simulink model "ABAG"  (R2015a)
settings: Solver=ode3  StartTime=0.0  StopTime=10.0  FixedStep=0.1  RelTol=1e-3
libraries: simulink x1
settings Model: Creator=s141010  LastModifiedBy=s141010

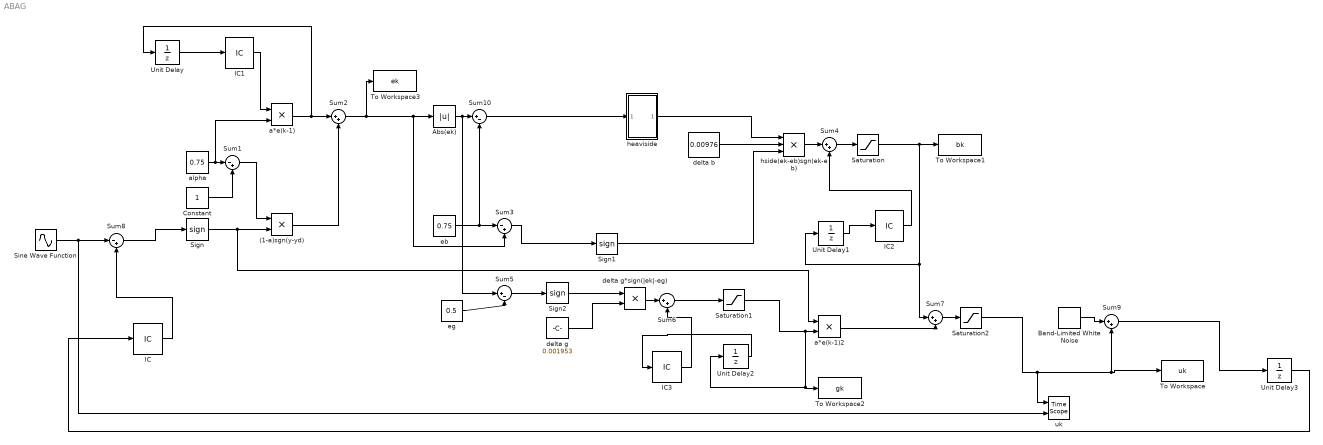
== system ABAG ==
  (1-a)sgn(y-yd) : Product
  Abs(ek) : Abs
  Band-Limited White Noise : simulink/Sources/Band-Limited White Noise  Cov=[0.1]  Ts=0.1  seed=[23341]
  Constant : Constant
  IC{,1..3} (4 alike) : InitialCondition
  Saturation : Saturate  UpperLimit=1  LowerLimit=0
  Saturation1 : Saturate  UpperLimit=1  LowerLimit=0
  Saturation2 : Saturate  UpperLimit=1  LowerLimit=0
  Sign : Signum
  Sign1 : Signum
  Sign2 : Signum
  Sine Wave Function : Sin  SampleTime=0.1
  Sum1 : Sum  Inputs=|-+
  Sum10 : Sum  Inputs=|+-
  Sum{2,4,6..7,9} (5 alike) : Sum  Inputs=|++
  Sum3 : Sum  Inputs=|-+
  Sum5 : Sum  Inputs=|+-
  Sum8 : Sum  Inputs=|-+
  To Workspace : ToWorkspace  VariableName=uk  SampleTime=-1
  To Workspace1 : ToWorkspace  VariableName=bk  SampleTime=-1
  To Workspace2 : ToWorkspace  VariableName=gk  SampleTime=-1
  To Workspace3 : ToWorkspace  VariableName=ek  SampleTime=-1
  Unit Delay : UnitDelay  InputProcessing=Columns as channels (frame based)  SampleTime=-1
  Unit Delay1 : UnitDelay  SampleTime=-1
  Unit Delay2 : UnitDelay  InputProcessing=Columns as channels (frame based)  SampleTime=-1
  Unit Delay3 : UnitDelay  SampleTime=-1
  a*e(k-1) : Product
  a*e(k-1)2 : Product
  alpha : Constant  Value=0.75
  delta b : Constant  Value=0.00976
  delta g : Constant  Value=0.001953
  delta g*sign(|ek|-eg) : Product
  eb : Constant  Value=0.75
  eg : Constant  Value=0.5
  heaviside : Subsystem
  hside(ek-eb)sgn(ek-eb) : Product  Inputs=3
  uk : TimeScope  NumInputPorts=2
  wires:
  Sign/1 -> a*e(k-1)2/1, (1-a)sgn(y-yd)/2
  Sum1/1 -> (1-a)sgn(y-yd)/1
  Constant/1 -> Sum1/2
  alpha/1 -> a*e(k-1)/2, Sum1/1
  (1-a)sgn(y-yd)/1 -> Sum2/2
  Sum2/1 -> To Workspace3/1, Abs(ek)/1, Sum3/2
  eb/1 -> Sum3/1, Sum10/2
  hside(ek-eb)sgn(ek-eb)/1 -> Sum4/1
  Saturation/1 -> To Workspace1/1, Sum7/1, Unit Delay1/1
  Sum3/1 -> Sign1/1
  eg/1 -> Sum5/2
  Sum5/1 -> Sign2/1
  Sign2/1 -> delta g*sign(|ek|-eg)/1
  delta g/1 -> delta g*sign(|ek|-eg)/2
  Unit Delay2/1 -> IC3/1
  delta g*sign(|ek|-eg)/1 -> Sum6/1
  Sine Wave Function/1 -> uk/2, Sum8/1
  Unit Delay3/1 -> IC/1
  Sum8/1 -> Sign/1
  Band-Limited White Noise/1 -> Sum9/1
  Sum9/1 -> Unit Delay3/1
  Sum4/1 -> Saturation/1
  Saturation1/1 -> Unit Delay2/1, To Workspace2/1, a*e(k-1)2/2
  Sum6/1 -> Saturation1/1
  Sum7/1 -> Saturation2/1
  Saturation2/1 -> To Workspace/1, Sum9/2, uk/1
  a*e(k-1)2/1 -> Sum7/2
  Sign1/1 -> hside(ek-eb)sgn(ek-eb)/3
  Abs(ek)/1 -> Sum5/1, Sum10/1
  a*e(k-1)/1 -> Unit Delay/1, Sum2/1
  Unit Delay1/1 -> IC2/1
  Sum10/1 -> heaviside/1(In1)
  heaviside/1(Out1) -> hside(ek-eb)sgn(ek-eb)/1
  delta b/1 -> hside(ek-eb)sgn(ek-eb)/2
  Unit Delay/1 -> IC1/1
  IC1/1 -> a*e(k-1)/1
  IC/1 -> Sum8/2
  IC2/1 -> Sum4/2
  IC3/1 -> Sum6/2

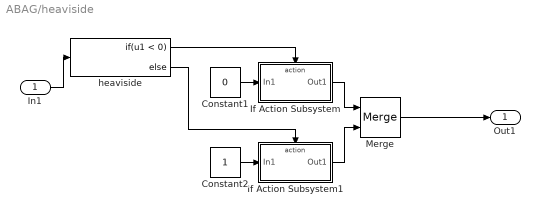
== system ABAG/heaviside ==
  In1 : Inport
  Constant1 : Constant  Value=0
  Constant2 : Constant
  If Action Subsystem : Subsystem  TreatAsAtomicUnit=on
  If Action Subsystem1 : Subsystem  TreatAsAtomicUnit=on
  Merge : Merge
  heaviside : If  IfExpression=u1 < 0
  Out1 : Outport
  wires:
  If Action Subsystem1/1(Out1) -> Merge/2
  Constant1/1 -> If Action Subsystem/1(In1)
  Constant2/1 -> If Action Subsystem1/1(In1)
  Merge/1 -> Out1/1
  If Action Subsystem/1(Out1) -> Merge/1
  heaviside/1 -> If Action Subsystem/Action
  heaviside/2 -> If Action Subsystem1/Action
  In1/1 -> heaviside/1

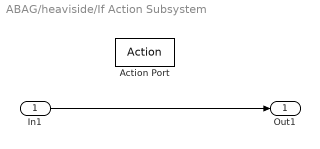
== system ABAG/heaviside/If Action Subsystem ==
  In1 : Inport
  Action Port : ActionPort  ActionType=then
  Out1 : Outport
  wires:
  In1/1 -> Out1/1

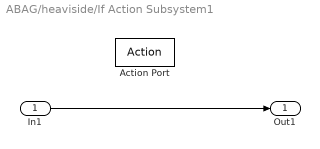
== system ABAG/heaviside/If Action Subsystem1 ==
  In1 : Inport
  Action Port : ActionPort  ActionType=else
  Out1 : Outport
  wires:
  In1/1 -> Out1/1
